simulink model "callGAMS"  (R2021b)
settings: Solver=ode1  StartTime=0.0  StopTime=20  FixedStep=1e-4  RelTol=1e-3
model workspace (MAT data in the model file):
  firstOrder = 60
  g2Max = 0
  runTime = 4
undefined symbols (not defined in the file or in its folder): c0, c1, D11, Delta, fg, G2gen, G3gen, G5gen, G6gen, G7gen, Iovc, l0, l1, Newton, r0, r1, Raphson, Rtpu, S1non, S2non, S3non, S5non, S6non, S7non, sigbuilder_block, tonvsc, Ts, Vhv, Vmv, w_pll, wc1, wdc1, wpq1, wsw1, Xtpu
libraries: simulink_extras x122, simulink x73, spsFirstOrderFilterLib x72, spsGroundLib x61, spsCurrentMeasurementLib x33, spsVoltageMeasurementLib x33, eeTransforms x24, spsabctoAlphaBetaZeroLib x12, spsControlledVoltageSourceLib x12, spsControlledCurrentSourceLib x12, spsPower3phPhasorLib x11, spsLoadFlowBusLib x9
(part 1 of 16)
Description:
  | Model of a simple control system for use iin training.
settings Model: SimulationMode=accelerator  PacingRate=0.100000  Creator=Paul Baracos  LastModifiedBy=oenoch
settings SolverCC: AlgebraicLoopSolver=TrustRegion
settings DataIOCC: LimitDataPoints=on  SaveOperatingPoint=on  SaveFormat=Array  SignalLoggingSaveFormat=ModelDataLogs  SaveOutput=off  SaveTime=off  ReturnWorkspaceOutputs=off  SignalLoggingName=sigsOut
settings OptimizationCC: BlockReduction=off  BooleanDataType=off  OptimizeBlockIOStorage=off  BufferReuse=off  GlobalBufferReuse=off  ExpressionFolding=off  LocalBlockOutputs=off  InitFltsAndDblsToZero=on  EfficientMapNaN2IntZero=off  LifeSpan=inf  OptimizeDataStoreBuffers=off  BusAssignmentInplaceUpdate=off
settings DebuggingCC: SaveWithParameterizedLinksMsg=none  UnderspecifiedInitializationDetection=Classic  MergeDetectMultiDrivingBlocksExec=none  SignalResolutionControl=TryResolveAllWithWarning  MultiTaskDSMMsg=warning  MultiTaskCondExecSysMsg=none  FcnCallInpInsideContextMsg=warning  UnconnectedInputMsg=none  UnconnectedOutputMsg=none  UnconnectedLineMsg=none  SFUnexpectedBacktrackingDiag=warning  SFNoUnconditionalDefaultTransitionDiag=warning  SFExecutionAtInitializationDiag=none  SFMachineParentedDataDiag=warning  ArithmeticOperatorsInVariantConditions=warning
settings HardwareCC: ProdBitPerPointer=32  ProdBitPerSizeT=32  ProdBitPerPtrDiffT=32  ProdLargestAtomicFloat=None  ProdIntDivRoundTo=Undefined  ProdEndianess=Unspecified  ProdWordSize=32  ProdHWDeviceType=32-bit Generic  TargetBitPerPointer=64  TargetBitPerSizeT=64  TargetBitPerPtrDiffT=64  TargetLongLongMode=on  TargetIntDivRoundTo=Zero  TargetEndianess=LittleEndian  TargetWordSize=64  TargetHWDeviceType=MATLAB Host  ProdEqTarget=off
settings ModelReferenceCC: PropagateSignalLabelsOutOfModel=off
settings SFSimCC: SimUseLocalCustomCode=off  CustomCodeUndefinedFunction=UseInterfaceOnly
settings CodeAppCC: MaxIdLength=128
settings GRTTargetCC: TargetLangStandard=C89/C90 (ANSI)  CombineOutputUpdateFcns=off  GRTInterface=on
settings ConfigComp: CovMetricSettings=dw  CovSaveCumulativeToWorkspaceVar=on  CovSaveSingleToWorkspaceVar=on  CovExternalEMLEnable=off

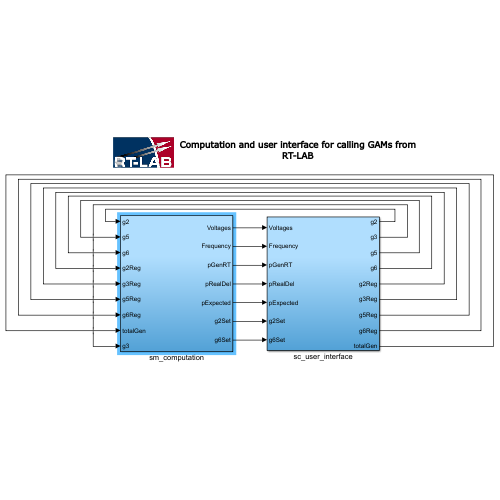
[thumbnail: Simulink's stored preview of the top-level diagram]
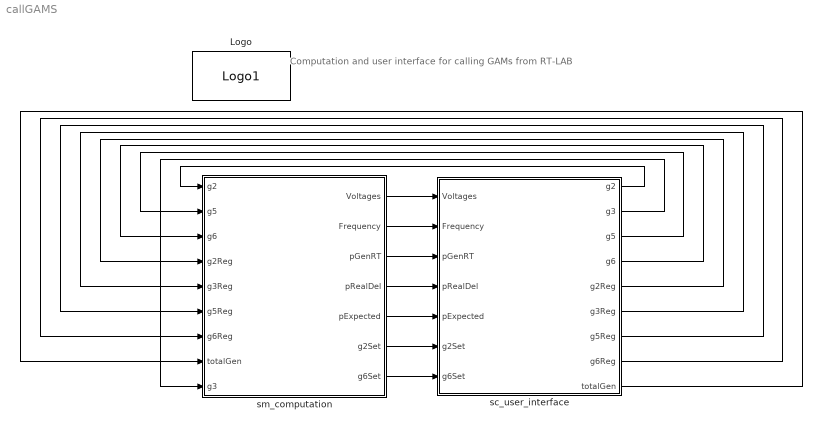
== system callGAMS ==
  note: Computation and user interface for calling GAMs from RT-LAB
  Logo : opal_lib/Logo1  vide=[]
  sc_user_interface : Subsystem
  sm_computation : Subsystem
  wires:
  sc_user_interface/1(g2) -> sm_computation/1(g2)
  sc_user_interface/2(g3) -> sm_computation/9(g3)
  sc_user_interface/3(g5) -> sm_computation/2(g5)
  sc_user_interface/4(g6) -> sm_computation/3(g6)
  sc_user_interface/5(g2Reg) -> sm_computation/4(g2Reg)
  sc_user_interface/6(g3Reg) -> sm_computation/5(g3Reg)
  sc_user_interface/7(g5Reg) -> sm_computation/6(g5Reg)
  sc_user_interface/8(g6Reg) -> sm_computation/7(g6Reg)
  sc_user_interface/9(totalGen) -> sm_computation/8(totalGen)
  sm_computation/1(Voltages) -> sc_user_interface/1(Voltages)
  sm_computation/2(Frequency) -> sc_user_interface/2(Frequency)
  sm_computation/3(pGenRT) -> sc_user_interface/3(pGenRT)
  sm_computation/4(pRealDel) -> sc_user_interface/4(pRealDel)
  sm_computation/5(pExpected) -> sc_user_interface/5(pExpected)
  sm_computation/6(g2Set) -> sc_user_interface/6(g2Set)
  sm_computation/7(g6Set) -> sc_user_interface/7(g6Set)

== system callGAMS/sc_user_interface ==
  note: Plots
  note: Input to the computation model
  note: Results from optimzation and dynamic model
  note: User interface: display acquisition signals and set control signals
  note: Real-time optimization
  Voltages : Inport
  Frequency : Inport  Port=2
  pGenRT : Inport  Port=3
  pRealDel : Inport  Port=4
  pExpected : Inport  Port=5
  g2Set : Inport  Port=6
  g6Set : Inport  Port=7
  Constant : Constant  OutMin=-10  OutMax=10
  Logo : opal_lib/Logo1  vide=[]
  OpComm : rtlab/OpComm  nbport=7  groupe_acq=1  subsys_rate=0  st=0  Synchronization=on  Interpolation=on  Threshold=1.0  Missed_Data=off  Sim_Time=off  Samples=off  dynSigOut=off  from_console=0  warning_done=off  writeOpCommFile=off  Offset=off
      settings: SourceProductName=RT-LAB
  Plots : Subsystem
  Pulse Generator : DiscretePulseGenerator  PulseType=Time based  Period=runTime  PulseWidth=5
  Pulse Generator1 : DiscretePulseGenerator  PulseType=Time based  Period=80  PulseWidth=5
  Real Time Redispatch Fn : Subsystem  TreatAsAtomicUnit=on
  Signal Builder : Subsystem  Tag=STV Subsys  Commented=on  LoadFcn=sigbuilder_block('load');  StartFcn=sigbuilder_block('start');  StopFcn=sigbuilder_block('stop');  ClipboardFcn=sigbuilder_block('clipboard');  mask(Sigbuilder block){tuvar=[0:10]}
      mask help: Simulink:masks:SigbuilderBlock_MD
      mask init:
      | if ~strcmp(get_param(bdroot(gcbh),'SimulationStatus'),'stopped') tuvar = sigbuilder_block('maskInit'); end
      settings: CopyFcn=sigbuilder_block('copy');  DeleteFcn=sigbuilder_block('delete');  ModelCloseFcn=sigbuilder_block('modelClose');  PreSaveFcn=sigbuilder_block('preSave');  PauseFcn=sigbuilder_block('pause');  ContinueFcn=sigbuilder_block('continue');  NameChangeFcn=sigbuilder_block('namechange');  OpenFcn=sigbuilder_block('open',[437.6 199.2 550.4 400 ]);  CloseFcn=sigbuilder_block('close');
      mask Display: plot(0, 0, 100, 100,[2, 2, 32, 32, 2], [68, 8, 8, 68, 68],[32, 2], [38, 38], [32, 19, 2],[53, 60, 44], [32, 17, 17, 2],[16, 16, 31, 31]);txt = getActiveGroup(gcbh);text(2, 100, txt,'verticalAlignment', 'top');
  TSO command : simulink/Math Operations/Slider Gain  gain=0  low=-50  high=50
  Triggered Subsystem : Subsystem  TreatAsAtomicUnit=on
  g2 : Outport
  g3 : Outport  Port=2
  g5 : Outport  Port=3
  g6 : Outport  Port=4
  g2Reg : Outport  Port=5
  g3Reg : Outport  Port=6
  g5Reg : Outport  Port=7
  g6Reg : Outport  Port=8
  totalGen : Outport  Port=9
  tag scope: freqs=global, g2Set=global, g6Set=global, voltages=global
  wires:
  TSO command/1 -> [tsoComm]
  Constant/1 -> TSO command/1
  [tsoComm] -> Real Time Redispatch Fn/1(tsoComm)
  Triggered Subsystem/1(Out1) -> Real Time Redispatch Fn/2(pGenRT)
  [pRealDel] -> Triggered Subsystem/2(In2)
  Triggered Subsystem/3(Output1) -> Real Time Redispatch Fn/4(gExpected)
  [pExpected] -> Triggered Subsystem/3(In3)
  Real Time Redispatch Fn/3(g5) -> g5/1, [g5]
  Triggered Subsystem/2(Output) -> Real Time Redispatch Fn/3(pPrev)
  Real Time Redispatch Fn/8(g6Reg) -> [g6Reg], g6Reg/1
  [pGenRT] -> Triggered Subsystem/1(In1)
  Real Time Redispatch Fn/2(g3) -> g3/1, [g3]
  Real Time Redispatch Fn/9(totalGen) -> [totalGen], totalGen/1
  Real Time Redispatch Fn/7(g5Reg) -> g5Reg/1
  Real Time Redispatch Fn/4(g6) -> g6/1, [g6]
  Real Time Redispatch Fn/6(g3Reg) -> g3Reg/1, [g3Reg]
  Pulse Generator/1 -> Real Time Redispatch Fn/Trigger
  Real Time Redispatch Fn/5(g2Reg) -> g2Reg/1, [g2Reg]
  Real Time Redispatch Fn/1(g2) -> g2/1, [g2]
  Pulse Generator1/1 -> Triggered Subsystem/Trigger
  Voltages/1 -> OpComm/1
  OpComm/1 -> [voltages]
  OpComm/2 -> [freqs]
  OpComm/3 -> [pGenRT]
  pGenRT/1 -> OpComm/3
  Frequency/1 -> OpComm/2
  pRealDel/1 -> OpComm/4
  pExpected/1 -> OpComm/5
  OpComm/4 -> [pRealDel]
  OpComm/5 -> [pExpected]
  g2Set/1 -> OpComm/6
  g6Set/1 -> OpComm/7
  OpComm/6 -> [g2Set]
  OpComm/7 -> [g6Set]

== system callGAMS/sm_computation ==
  note: Dynamic model
  note: Computation is done in this subsystem
  note: Results from optimzation and dynamic model
  g2 : Inport
  g5 : Inport  Port=2
  g6 : Inport  Port=3
  g2Reg : Inport  Port=4
  g3Reg : Inport  Port=5
  g5Reg : Inport  Port=6
  g6Reg : Inport  Port=7
  totalGen : Inport  Port=8
  g3 : Inport  Port=9
  B1 : Subsystem
  B2 : Subsystem
  B3 : Subsystem
  B4 : Subsystem
  B5 : Subsystem
  B6 : Subsystem
  B7 : Subsystem
  G1 : Subsystem
      mask Display:
      | disp('SG')
      | %x = [0:0.001:1];
      | %y = 0.2*sin(10*x) + 0.5;
      | %plot(x,y)
  G2 : Subsystem
  G2s : spsThreePhaseSourceLib/Three-Phase Source  Commented=on  InternalConnection=Yg  VoltagePhases=off  Voltage=(220000)*1.02346  PhaseAngle=-22.8275  Voltage_phases=[25e3 25e3 25e3]/sqrt(3)  PhaseAngles_phases=[0 -120 +120]  Frequency=fg  NonIdealSource=on  SpecifyImpedance=off  Resistance=Rtpu*(Vhv^2/S2non)  Inductance=Xtpu*(Vhv^2/S3non) * 1/(2*pi*fg)  ShortCircuitLevel=100e6  BaseVoltage=Vhv  XRratio=7  BusType=PQ  Pref=45000000  Qref=5000000  Prefabc=[10e3, 10e3, 10e3]  Qrefabc=[0, 0, 0]  Qmin=-inf  Qmax=inf
  G3 : Subsystem
  G3s : spsThreePhaseSourceLib/Three-Phase Source  Commented=on  InternalConnection=Yg  VoltagePhases=off  Voltage=(220000)*1.02196  PhaseAngle=-23.0407  Voltage_phases=[25e3 25e3 25e3]/sqrt(3)  PhaseAngles_phases=[0 -120 +120]  Frequency=fg  NonIdealSource=on  SpecifyImpedance=off  Resistance=Rtpu*(Vhv^2/S3non)  Inductance=Xtpu*(Vhv^2/S3non) * 1/(2*pi*fg)  ShortCircuitLevel=100e6  BaseVoltage=Vhv  XRratio=7  BusType=PQ  Pref=45000000  Qref=5000000  Prefabc=[10e3, 10e3, 10e3]  Qrefabc=[0, 0, 0]  Qmin=-inf  Qmax=inf
  G5 : Subsystem
  G5s : spsThreePhaseSourceLib/Three-Phase Source  Commented=on  InternalConnection=Yg  VoltagePhases=off  Voltage=(220000)*1.02214  PhaseAngle=-22.9944  Voltage_phases=[25e3 25e3 25e3]/sqrt(3)  PhaseAngles_phases=[0 -120 +120]  Frequency=fg  NonIdealSource=on  SpecifyImpedance=off  Resistance=Rtpu*(Vhv^2/S5non)  Inductance=Xtpu*(Vhv^2/S5non) * 1/(2*pi*fg)  ShortCircuitLevel=100e6  BaseVoltage=Vhv  XRratio=7  BusType=PQ  Pref=45000000  Qref=5000000  Prefabc=[10e3, 10e3, 10e3]  Qrefabc=[0, 0, 0]  Qmin=-inf  Qmax=inf
  G6 : Subsystem
  G6s : spsThreePhaseSourceLib/Three-Phase Source  Commented=on  InternalConnection=Yg  VoltagePhases=off  Voltage=(220000)*1.02275  PhaseAngle=-22.9111  Voltage_phases=[25e3 25e3 25e3]/sqrt(3)  PhaseAngles_phases=[0 -120 +120]  Frequency=fg  NonIdealSource=on  SpecifyImpedance=off  Resistance=Rtpu*(Vhv^2/S6non)  Inductance=Xtpu*(Vhv^2/S6non) * 1/(2*pi*fg)  ShortCircuitLevel=100e6  BaseVoltage=Vhv  XRratio=7  BusType=PQ  Pref=45000000  Qref=5000000  Prefabc=[10e3, 10e3, 10e3]  Qrefabc=[0, 0, 0]  Qmin=-inf  Qmax=inf
  G7 : Subsystem
      mask Display:
      | disp('SG')
      | %x = [0:0.001:1];
      | %y = 0.2*sin(10*x) + 0.5;
      | %plot(x,y)
  Logo : opal_lib/Logo1  vide=[]
  Measurements EMT : Subsystem  Commented=on
  Measurements Phasor : Subsystem
  OpComm : rtlab/OpComm  nbport=9  groupe_acq=1  subsys_rate=0  st=0  Synchronization=on  Interpolation=on  Threshold=1.0  Missed_Data=off  Sim_Time=off  Samples=off  dynSigOut=off  from_console=1  warning_done=off  writeOpCommFile=off  Offset=off
      settings: SourceProductName=RT-LAB
  Three-Phase PI Section Line{1,3,7,10} (4 alike) : spsThreePhasePISectionLineLib/Three-Phase PI Section Line  LConnTagsString=a|b|c  RConnTagsString=A|B|C  Length=20  Frequency=fg  Resistances=[r1 r0]  Inductances="[l1  l0]"  Capacitances=[c1 c0]
  Three-Phase PI Section Line2 : spsThreePhasePISectionLineLib/Three-Phase PI Section Line  LConnTagsString=a|b|c  RConnTagsString=A|B|C  Length=40  Frequency=fg  Resistances=[r1 r0]  Inductances="[l1  l0]"  Capacitances=[c1 c0]
  Three-Phase PI Section Line4 : spsThreePhasePISectionLineLib/Three-Phase PI Section Line  LConnTagsString=a|b|c  RConnTagsString=A|B|C  Length=10  Frequency=fg  Resistances=[r1 r0]  Inductances="[l1  l0]"  Capacitances=[c1 c0]
  Three-Phase PI Section Line5 : spsThreePhasePISectionLineLib/Three-Phase PI Section Line  LConnTagsString=a|b|c  RConnTagsString=A|B|C  Length=30  Frequency=fg  Resistances=[r1 r0]  Inductances="[l1  l0]"  Capacitances=[c1 c0]
  Three-Phase PI Section Line9 : spsThreePhasePISectionLineLib/Three-Phase PI Section Line  LConnTagsString=a|b|c  RConnTagsString=A|B|C  Length=10  Frequency=fg  Resistances=[r1 r0]  Inductances="[l1  l0]"  Capacitances=[c1 c0]
  Three-Phase Parallel RLC Load1 : spsThreePhaseParallelRLCLoadLib/Three-Phase Parallel RLC Load  LConnTagsString=A|B|C  Configuration=Y (grounded)  NominalVoltage=Vhv  Vabc=[1e3 1e3 1e3]  Vabcp=[1e3 1e3 1e3]  NominalFrequency=fg  UnbalancedPower=off  ActivePower=81750000  InductivePower=10196203.4628  CapacitivePower=0  Pabc=[10e3 9e3 11e3]  QLabc=[100 90 110]  QCabc=[100 90 110]  Pabcp=[10e3 9e3 11e3]  QLabcp=[100 90 110]  QCabcp=[100 90 110]  Measurements=None  LoadType=constant Z
  Three-Phase Parallel RLC Load2 : spsThreePhaseParallelRLCLoadLib/Three-Phase Parallel RLC Load  LConnTagsString=A|B|C  Configuration=Y (grounded)  NominalVoltage=Vhv  Vabc=[1e3 1e3 1e3]  Vabcp=[1e3 1e3 1e3]  NominalFrequency=fg  UnbalancedPower=off  ActivePower=115375000  InductivePower=20395570.7066  CapacitivePower=0  Pabc=[10e3 9e3 11e3]  QLabc=[100 90 110]  QCabc=[100 90 110]  Pabcp=[10e3 9e3 11e3]  QLabcp=[100 90 110]  QCabcp=[100 90 110]  Measurements=None  LoadType=constant Z
  Three-Phase Parallel RLC Load3 : spsThreePhaseParallelRLCLoadLib/Three-Phase Parallel RLC Load  LConnTagsString=A|B|C  Configuration=Y (grounded)  NominalVoltage=Vhv  Vabc=[1e3 1e3 1e3]  Vabcp=[1e3 1e3 1e3]  NominalFrequency=fg  UnbalancedPower=off  ActivePower=47250000  InductivePower=5398734.4876  CapacitivePower=0  Pabc=[10e3 9e3 11e3]  QLabc=[100 90 110]  QCabc=[100 90 110]  Pabcp=[10e3 9e3 11e3]  QLabcp=[100 90 110]  QCabcp=[100 90 110]  Measurements=None  LoadType=constant Z
  Three-Phase Parallel RLC Load6 : spsThreePhaseParallelRLCLoadLib/Three-Phase Parallel RLC Load  LConnTagsString=A|B|C  Configuration=Y (grounded)  NominalVoltage=Vhv  Vabc=[1e3 1e3 1e3]  Vabcp=[1e3 1e3 1e3]  NominalFrequency=fg  UnbalancedPower=off  ActivePower=47250000  InductivePower=10398734.4876  CapacitivePower=0  Pabc=[10e3 9e3 11e3]  QLabc=[100 90 110]  QCabc=[100 90 110]  Pabcp=[10e3 9e3 11e3]  QLabcp=[100 90 110]  QCabcp=[100 90 110]  Measurements=None  LoadType=constant Z
  Three-Phase Parallel RLC Load7 : spsThreePhaseParallelRLCLoadLib/Three-Phase Parallel RLC Load  LConnTagsString=A|B|C  Configuration=Y (grounded)  NominalVoltage=Vhv  Vabc=[1e3 1e3 1e3]  Vabcp=[1e3 1e3 1e3]  NominalFrequency=fg  UnbalancedPower=off  ActivePower=20875000  InductivePower=5598101.7314  CapacitivePower=0  Pabc=[10e3 9e3 11e3]  QLabc=[100 90 110]  QCabc=[100 90 110]  Pabcp=[10e3 9e3 11e3]  QLabcp=[100 90 110]  QCabcp=[100 90 110]  Measurements=None  LoadType=constant Z
  powergui : spspowerguiLib/powergui  Priority=1  SimulationMode=Phasor  SampleTime=50e-6  frequency=fg  Iterations=50  frequencyindice=50  Pbase=100e6  ErrMax=0.0001  UnitsV=kV  UnitsW=MW  buscounter=0  FunctionMessages=off  echomessages=off  EnableUseOfTLC=off  CurrentSourceSwitches=off  DisableSnubberDevices=off  DisableRonSwitches=off  DisableVfSwitches=off  DisplayEquations=off  AutomaticDiscreteSolvers=off  SolverType=Tustin/Backward Euler (TBE)  Interpol=off  ExternalGateDelay=off  methode=off  Ts=100  x0status=blocks  SPID=on  SwTol=0  HookPort=off  NonlinearTolerance=1e-4  nMaxIteration=100  ContinueOnMaxIteration=off  RestoreLinks=warning  ResistiveCurrentMeasurement=off  Frange=[0:2:500]  Ylog=off  Xlog=on  ShowGrid=off  save=off  variable=ZData  structure=0  ZoomFFT=off  StartTime=0.0  cycles=1  DisplayStyle=1  fundamental=60  FreqAxis=off  MaxFrequency=1000  frequencyindicesteady=1  RmsSteady=1  display=off
  Voltages : Outport
  Frequency : Outport  Port=2
  pGenRT : Outport  Port=3
  pRealDel : Outport  Port=4  VectorParamsAs1DForOutWhenUnconnected=off
  pExpected : Outport  Port=5  VectorParamsAs1DForOutWhenUnconnected=off
  g2Set : Outport  Port=6  VectorParamsAs1DForOutWhenUnconnected=off
  g6Set : Outport  Port=7  VectorParamsAs1DForOutWhenUnconnected=off
  tag scope: g2=global, g2Reg=global, g3=global, g3Reg=global, g5=global, g5Reg=global, g6=global, g6Reg=global, totalGen=global
  wires:
  Measurements Phasor/1(Voltages) -> Voltages/1
  Measurements Phasor/2(Frequency) -> Frequency/1
  totalGen/1 -> OpComm/9
  g6Reg/1 -> OpComm/8
  g5Reg/1 -> OpComm/7
  g3Reg/1 -> OpComm/6
  g2Reg/1 -> OpComm/5
  g6/1 -> OpComm/4
  g5/1 -> OpComm/3
  g2/1 -> OpComm/1
  g3/1 -> OpComm/2
  OpComm/1 -> [g2]
  OpComm/5 -> [g2Reg]
  OpComm/2 -> [g3]
  OpComm/3 -> [g5]
  OpComm/4 -> [g6]
  OpComm/6 -> [g3Reg]
  OpComm/7 -> [g5Reg]
  OpComm/8 -> [g6Reg]
  OpComm/9 -> [totalGen]
  Measurements Phasor/3(pGenRT) -> pGenRT/1
  Measurements Phasor/4(pRealDel) -> pRealDel/1
  Measurements Phasor/5(pExpected) -> pExpected/1
  G2/1(Output) -> g2Set/1
  G6/1(Output) -> g6Set/1
  connections:
  Three-Phase PI Section Line1/LConn1 -- B2/RConn1 -- Three-Phase PI Section Line7/LConn1
  B5/RConn3 -- Three-Phase PI Section Line5/LConn3 -- Three-Phase PI Section Line7/RConn3 -- Three-Phase PI Section Line3/LConn3 -- Three-Phase PI Section Line4/LConn3 -- Three-Phase Parallel RLC Load2/LConn3
  Three-Phase Parallel RLC Load7/LConn1 -- Three-Phase PI Section Line10/RConn1 -- Three-Phase PI Section Line3/RConn1 -- B6/LConn1
  Three-Phase Parallel RLC Load3/LConn1 -- B7/LConn1 -- Three-Phase PI Section Line5/RConn1
  B4/RConn1 -- Three-Phase PI Section Line9/LConn1 -- Three-Phase PI Section Line10/LConn1 -- Three-Phase PI Section Line2/RConn1
  Three-Phase PI Section Line9/RConn2 -- B3/LConn2 -- Three-Phase Parallel RLC Load6/LConn2
  Three-Phase Parallel RLC Load7/LConn2 -- Three-Phase PI Section Line10/RConn2 -- Three-Phase PI Section Line3/RConn2 -- B6/LConn2
  Three-Phase PI Section Line9/RConn1 -- B3/LConn1 -- Three-Phase Parallel RLC Load6/LConn1
  Three-Phase Parallel RLC Load3/LConn3 -- B7/LConn3 -- Three-Phase PI Section Line5/RConn3
  B6/RConn2 -- G6s/RConn2 -- G6/RConn2
  B5/RConn1 -- Three-Phase PI Section Line5/LConn1 -- Three-Phase PI Section Line7/RConn1 -- Three-Phase PI Section Line3/LConn1 -- Three-Phase PI Section Line4/LConn1 -- Three-Phase Parallel RLC Load2/LConn1
  Three-Phase PI Section Line1/LConn3 -- B2/RConn3 -- Three-Phase PI Section Line7/LConn3
  B3/RConn2 -- G3s/RConn2 -- G3/RConn2
  B5/RConn2 -- Three-Phase PI Section Line5/LConn2 -- Three-Phase PI Section Line7/RConn2 -- Three-Phase PI Section Line3/LConn2 -- Three-Phase PI Section Line4/LConn2 -- Three-Phase Parallel RLC Load2/LConn2
  B6/RConn3 -- G6s/RConn3 -- G6/RConn3
  Three-Phase Parallel RLC Load1/LConn2 -- B4/LConn2 -- Three-Phase PI Section Line4/RConn2 -- Three-Phase PI Section Line1/RConn2
  B3/RConn1 -- G3s/RConn1 -- G3/RConn1
  B3/RConn3 -- G3s/RConn3 -- G3/RConn3
  Three-Phase Parallel RLC Load1/LConn1 -- B4/LConn1 -- Three-Phase PI Section Line4/RConn1 -- Three-Phase PI Section Line1/RConn1
  Three-Phase Parallel RLC Load3/LConn2 -- B7/LConn2 -- Three-Phase PI Section Line5/RConn2
  Three-Phase PI Section Line9/RConn3 -- B3/LConn3 -- Three-Phase Parallel RLC Load6/LConn3
  B6/RConn1 -- G6s/RConn1 -- G6/RConn1
  Three-Phase PI Section Line1/LConn2 -- B2/RConn2 -- Three-Phase PI Section Line7/LConn2
  B2/LConn3 -- G2s/RConn3 -- G2/RConn3
  B2/LConn1 -- G2s/RConn1 -- G2/RConn1
  Three-Phase Parallel RLC Load7/LConn3 -- Three-Phase PI Section Line10/RConn3 -- Three-Phase PI Section Line3/RConn3 -- B6/LConn3
  Three-Phase Parallel RLC Load1/LConn3 -- B4/LConn3 -- Three-Phase PI Section Line4/RConn3 -- Three-Phase PI Section Line1/RConn3
  Three-Phase PI Section Line2/LConn3 -- B1/RConn3
  Three-Phase PI Section Line2/LConn1 -- B1/RConn1
  G1/RConn1 -- B1/LConn1
  G1/RConn2 -- B1/LConn2
  Three-Phase PI Section Line2/LConn2 -- B1/RConn2
  G1/RConn3 -- B1/LConn3
  G7/RConn1 -- B7/RConn1
  G7/RConn2 -- B7/RConn2
  G7/RConn3 -- B7/RConn3
  B4/RConn3 -- Three-Phase PI Section Line10/LConn3 -- Three-Phase PI Section Line9/LConn3 -- Three-Phase PI Section Line2/RConn3
  B4/RConn2 -- Three-Phase PI Section Line2/RConn2 -- Three-Phase PI Section Line9/LConn2 -- Three-Phase PI Section Line10/LConn2
  G5s/RConn3 -- G5/RConn3 -- B5/LConn3
  G5/RConn1 -- G5s/RConn1 -- B5/LConn1
  G2s/RConn2 -- B2/LConn2 -- G2/RConn2
  G5/RConn2 -- B5/LConn2 -- G5s/RConn2

== system callGAMS/sc_user_interface/Plots ==
  note: Multiple commands
  note: System parameters
  note: Individual active power generation and regulation of VPP units
  note: Total active power generation from Pset,
      | units and dynamic model
  All o/p scope : Scope
  Frequency scope : Scope
  From10 : From  Commented=on  GotoTag=g2Set
  From12 : From  Commented=on  GotoTag=g3Set
  From13 : From  Commented=on  GotoTag=g5Set
  From29 : From  Commented=on  GotoTag=g6Set
  Gain : Gain  Gain=1/100
  Gain1 : Gain  Gain=1/100
  Gain2 : Gain  Gain=1e6
  Generation and Regulation scope : Scope
  Goto3 : Goto  Commented=on  GotoTag=pSet  TagVisibility=global
  Integrator : Integrator  InitialCondition=S2non*G2gen
  Integrator1 : Integrator  InitialCondition=S6non*G6gen
  Mux : Mux  Inputs=2
  Mux1 : Mux  Inputs=8
  Mux10 : Mux  Inputs=2
  Mux6 : Mux  Commented=on
  Mux8 : Mux
  Mux9 : Mux
  Power scope : Scope
  Sum : Sum  Inputs=|+-
  Sum of Elements : Sum  Commented=on  Inputs=+
  Sum1 : Sum  Inputs=|+-
  Sum2 : Sum  Inputs=+-+-
  To Workspace : ToWorkspace  VariableName=pGoutWpp  SaveFormat=Structure With Time  SampleTime=-1
  To Workspace1 : ToWorkspace  VariableName=pGoutPv  SaveFormat=Structure With Time  SampleTime=-1
  To Workspace2 : ToWorkspace  VariableName=pMultiple  SaveFormat=Structure With Time  SampleTime=-1
  Voltage scope : Scope
  g2 scope1 : Scope  NumInputPorts=2
  g2 scope2 : Scope
  wires:
  [g2] -> Mux1/1
  [g5P] -> Mux1/3
  [g6P] -> Mux1/4
  [g2RegP] -> Mux1/5
  [pGenRT] -> Power scope/1
  [voltages] -> Voltage scope/1
  [freqs] -> Frequency scope/1
  From10/1 -> Mux6/3
  From12/1 -> Mux6/2
  [pSet] -> Mux/1  "pSet"
  From13/1 -> Mux6/1
  Mux/1 -> All o/p scope/1
  Mux1/1 -> Generation and Regulation scope/1
  [activePowerSum] -> Mux/2  "dynamic"
  [g5RegP] -> Mux1/7
  [g6RegP] -> Mux1/8
  From29/1 -> Mux6/4
  Mux6/1 -> Goto3/1, Sum of Elements/1
  Mux8/1 -> g2 scope1/1, To Workspace/1
  [g2Actual] -> Mux8/1  "Normal offer"
  [g2Set] -> Mux8/3  "gSet"
  Gain/1 -> Integrator/1
  Sum/1 -> Gain/1
  Integrator/1 -> Sum/2, Mux8/4  "First order 100secs"
  [g2Expected] -> Mux8/2, Sum/1  "Ex s"
  [g6Expected] -> Mux9/2, Sum1/1
  Sum1/1 -> Gain1/1
  Gain1/1 -> Integrator1/1
  [g6Actual] -> Mux9/1
  Integrator1/1 -> Mux9/4, Sum1/2  "First order 100secs"
  [g6Set] -> Mux9/3
  Mux9/1 -> g2 scope1/2, To Workspace1/1
  [tsoComm] -> Gain2/1
  Mux10/1 -> g2 scope2/1, To Workspace2/1
  [g2Set] -> Sum2/1  "gSet"
  [g6Set] -> Sum2/3  "gSet"
  [g2Actual] -> Sum2/2
  [g6Actual] -> Sum2/4
  Sum2/1 -> [rEff]
  [rEff] -> Mux10/2
  Gain2/1 -> Mux10/1

== system callGAMS/sc_user_interface/Real Time Redispatch Fn ==
  tsoComm : Inport
  pGenRT : Inport  Port=2
  pPrev : Inport  Port=3
  gExpected : Inport  Port=4
  Trigger : TriggerPort  VariantControl=(inherit)
  MATLAB Function : MATLAB Function  TreatAsAtomicUnit=on
  g2 : Outport
  g3 : Outport  Port=2
  g5 : Outport  Port=3
  g6 : Outport  Port=4
  g2Reg : Outport  Port=5
  g3Reg : Outport  Port=6
  g5Reg : Outport  Port=7
  g6Reg : Outport  Port=8
  totalGen : Outport  Port=9
  wires:
  MATLAB Function/7(g5Reg) -> g5Reg/1
  MATLAB Function/6(g3Reg) -> g3Reg/1
  MATLAB Function/1(g2) -> g2/1
  MATLAB Function/4(g6) -> g6/1
  MATLAB Function/5(g2Reg) -> g2Reg/1
  MATLAB Function/3(g5) -> g5/1
  MATLAB Function/2(g3) -> g3/1
  tsoComm/1 -> MATLAB Function/1(tsoComm)
  pGenRT/1 -> MATLAB Function/2(pGenRT)
  pPrev/1 -> MATLAB Function/3(pPrev)
  gExpected/1 -> MATLAB Function/4(pExpected)
  MATLAB Function/8(g6Reg) -> g6Reg/1
  MATLAB Function/9(totalGen) -> totalGen/1

== system callGAMS/sc_user_interface/Signal Builder ==
  Demux : Demux  Tag=STV Demux  Outputs=1
      settings: DisplayOption=none
  FromWs : FromWorkspace  Tag=STV FromWs  VariableName=tuvar
      SigBuilderData=|
      | common.afterFinalStr = 'Extrapolate'
      | common.sampleTime = 0
      | dataSet.timeRange = [0 10]
      | dataSet.name = 'Group 1'
      | sbobj.Groups.Name = 'Group 1'
      | sbobj.Groups.Signals.Name = 'Signal 1'
      | sbobj.Groups.Signals.XData = [0 4 4 6 6 10]
      | sbobj.Groups.Signals.YData = [0 0 1 1 0 0]
  Signal 1 : Outport  Tag=STV Outport
  wires:
  Demux/1 -> Signal 1/1
  FromWs/1 -> Demux/1

== system callGAMS/sc_user_interface/Triggered Subsystem ==
  In1 : Inport  LatchByDelayingOutsideSignal=on
  In2 : Inport  Port=2  LatchByDelayingOutsideSignal=on
  In3 : Inport  Port=3  LatchByDelayingOutsideSignal=on
  Trigger : TriggerPort  VariantControl=(inherit)
  Out1 : Outport
  Output : Outport  Port=2
  Output1 : Outport  Port=3
  wires:
  In1/1 -> Out1/1
  In2/1 -> Output/1
  In3/1 -> Output1/1

== system callGAMS/sm_computation/B1 ==
  Current Measurement1 : spsCurrentMeasurementLib/Current Measurement  PhasorSimulation=on  OutputType=Complex  PSBequivalent=0
  Current Measurement2 : spsCurrentMeasurementLib/Current Measurement  PhasorSimulation=on  OutputType=Complex  PSBequivalent=0
  Current Measurement3 : spsCurrentMeasurementLib/Current Measurement  PhasorSimulation=on  OutputType=Complex  PSBequivalent=0
  Gain : Gain
  Gain1 : Gain
  Ground1 : spsGroundLib/Ground  LConnTagsString=a
  Ground2 : spsGroundLib/Ground  LConnTagsString=a
  Ground3 : spsGroundLib/Ground  LConnTagsString=a
  Load Flow Bus1 : spsLoadFlowBusLib/Load Flow Bus  LConnTagsString=a  Phases=single  Connectors=on one side  ID=B1  Vbase=Vhv  Vref=1  Vangle=0  VLF=1  VLFb=1  VLFc=1  angleLF=-30.01  angleLFb=0  angleLFc=0
      settings: SourceProductBaseCode=PS
  Mux : Mux  Inputs=3
  Mux1 : Mux  Inputs=3
  Voltage Measurement1 : spsVoltageMeasurementLib/Voltage Measurement  PhasorSimulation=on  OutputType=Complex  PSBequivalent=0
  Voltage Measurement2 : spsVoltageMeasurementLib/Voltage Measurement  PhasorSimulation=on  OutputType=Complex  PSBequivalent=0
  Voltage Measurement3 : spsVoltageMeasurementLib/Voltage Measurement  PhasorSimulation=on  OutputType=Complex  PSBequivalent=0
  A : PMIOPort  Side=Left
  B : PMIOPort  Port=2  Side=Left
  C : PMIOPort  Port=3  Side=Left
  a : PMIOPort  Port=4  Side=Right
  b : PMIOPort  Port=5  Side=Right
  c : PMIOPort  Port=6  Side=Right
  tag scope: Ig1=global, Vg1=global
  wires:
  Voltage Measurement2/1 -> Mux/3
  Voltage Measurement1/1 -> Mux/2
  Voltage Measurement3/1 -> Mux/1
  Current Measurement3/1 -> Mux1/1
  Current Measurement1/1 -> Mux1/2
  Current Measurement2/1 -> Mux1/3
  Mux/1 -> Gain/1
  Gain/1 -> [Vg1]
  Mux1/1 -> Gain1/1
  Gain1/1 -> [Ig1]
  connections:
  Current Measurement3/RConn1 -- a/RConn1
  B/RConn1 -- Current Measurement1/LConn1 -- Voltage Measurement1/LConn1
  C/RConn1 -- Current Measurement2/LConn1 -- Voltage Measurement2/LConn1
  Current Measurement3/LConn1 -- Voltage Measurement3/LConn1 -- Load Flow Bus1/LConn1 -- A/RConn1
  Current Measurement1/RConn1 -- b/RConn1
  Current Measurement2/RConn1 -- c/RConn1
  Ground3/LConn1 -- Voltage Measurement3/LConn2
  Ground1/LConn1 -- Voltage Measurement1/LConn2
  Ground2/LConn1 -- Voltage Measurement2/LConn2

== system callGAMS/sm_computation/B2 ==
  Current Measurement1 : spsCurrentMeasurementLib/Current Measurement  PhasorSimulation=on  OutputType=Complex  PSBequivalent=0
  Current Measurement2 : spsCurrentMeasurementLib/Current Measurement  PhasorSimulation=on  OutputType=Complex  PSBequivalent=0
  Current Measurement3 : spsCurrentMeasurementLib/Current Measurement  PhasorSimulation=on  OutputType=Complex  PSBequivalent=0
  Gain : Gain
  Gain1 : Gain
  Ground1 : spsGroundLib/Ground  LConnTagsString=a
  Ground2 : spsGroundLib/Ground  LConnTagsString=a
  Ground3 : spsGroundLib/Ground  LConnTagsString=a
  Load Flow Bus1 : spsLoadFlowBusLib/Load Flow Bus  LConnTagsString=a  Phases=single  Connectors=on one side  ID=B2  Vbase=Vhv  Vref=1  Vangle=0  VLF=0.9961  VLFb=1  VLFc=1  angleLF=-30.42  angleLFb=0  angleLFc=0
      settings: SourceProductBaseCode=PS
  Mux : Mux  Inputs=3
  Mux1 : Mux  Inputs=3
  Voltage Measurement1 : spsVoltageMeasurementLib/Voltage Measurement  PhasorSimulation=on  OutputType=Complex  PSBequivalent=0
  Voltage Measurement2 : spsVoltageMeasurementLib/Voltage Measurement  PhasorSimulation=on  OutputType=Complex  PSBequivalent=0
  Voltage Measurement3 : spsVoltageMeasurementLib/Voltage Measurement  PhasorSimulation=on  OutputType=Complex  PSBequivalent=0
  A : PMIOPort  Side=Left
  B : PMIOPort  Port=2  Side=Left
  C : PMIOPort  Port=3  Side=Left
  a : PMIOPort  Port=4  Side=Right
  b : PMIOPort  Port=5  Side=Right
  c : PMIOPort  Port=6  Side=Right
  tag scope: Ig2=global, Vg2=global
  wires:
  Voltage Measurement2/1 -> Mux/3
  Voltage Measurement1/1 -> Mux/2
  Voltage Measurement3/1 -> Mux/1
  Current Measurement3/1 -> Mux1/1
  Current Measurement1/1 -> Mux1/2
  Current Measurement2/1 -> Mux1/3
  Mux/1 -> Gain/1
  Gain/1 -> [Vg2]
  Mux1/1 -> Gain1/1
  Gain1/1 -> [Ig2]
  connections:
  Current Measurement3/RConn1 -- a/RConn1
  Voltage Measurement1/LConn1 -- B/RConn1 -- Current Measurement1/LConn1
  Voltage Measurement2/LConn1 -- C/RConn1 -- Current Measurement2/LConn1
  Voltage Measurement3/LConn1 -- Load Flow Bus1/LConn1 -- A/RConn1 -- Current Measurement3/LConn1
  Current Measurement1/RConn1 -- b/RConn1
  Current Measurement2/RConn1 -- c/RConn1
  Ground3/LConn1 -- Voltage Measurement3/LConn2
  Ground1/LConn1 -- Voltage Measurement1/LConn2
  Ground2/LConn1 -- Voltage Measurement2/LConn2

== system callGAMS/sm_computation/B3 ==
  Current Measurement1 : spsCurrentMeasurementLib/Current Measurement  PhasorSimulation=on  OutputType=Complex  PSBequivalent=0
  Current Measurement2 : spsCurrentMeasurementLib/Current Measurement  PhasorSimulation=on  OutputType=Complex  PSBequivalent=0
  Current Measurement3 : spsCurrentMeasurementLib/Current Measurement  PhasorSimulation=on  OutputType=Complex  PSBequivalent=0
  Gain : Gain
  Gain1 : Gain
  Ground1 : spsGroundLib/Ground  LConnTagsString=a
  Ground2 : spsGroundLib/Ground  LConnTagsString=a
  Ground3 : spsGroundLib/Ground  LConnTagsString=a
  Load Flow Bus1 : spsLoadFlowBusLib/Load Flow Bus  LConnTagsString=a  Phases=single  Connectors=on one side  ID=B3  Vbase=Vhv  Vref=1  Vangle=0  VLF=0.9945  VLFb=1  VLFc=1  angleLF=-30.65  angleLFb=0  angleLFc=0
      settings: SourceProductBaseCode=PS
  Mux : Mux  Inputs=3
  Mux1 : Mux  Inputs=3
  Voltage Measurement1 : spsVoltageMeasurementLib/Voltage Measurement  PhasorSimulation=on  OutputType=Complex  PSBequivalent=0
  Voltage Measurement2 : spsVoltageMeasurementLib/Voltage Measurement  PhasorSimulation=on  OutputType=Complex  PSBequivalent=0
  Voltage Measurement3 : spsVoltageMeasurementLib/Voltage Measurement  PhasorSimulation=on  OutputType=Complex  PSBequivalent=0
  A : PMIOPort  Side=Left
  B : PMIOPort  Port=2  Side=Left
  C : PMIOPort  Port=3  Side=Left
  a : PMIOPort  Port=4  Side=Right
  b : PMIOPort  Port=5  Side=Right
  c : PMIOPort  Port=6  Side=Right
  tag scope: Ig3=global, Vg3=global
  wires:
  Voltage Measurement2/1 -> Mux/3
  Voltage Measurement1/1 -> Mux/2
  Voltage Measurement3/1 -> Mux/1
  Current Measurement3/1 -> Mux1/1
  Current Measurement1/1 -> Mux1/2
  Current Measurement2/1 -> Mux1/3
  Mux/1 -> Gain/1
  Gain/1 -> [Vg3]
  Mux1/1 -> Gain1/1
  Gain1/1 -> [Ig3]
  connections:
  Current Measurement3/RConn1 -- a/RConn1
  Voltage Measurement1/LConn1 -- B/RConn1 -- Current Measurement1/LConn1
  Voltage Measurement2/LConn1 -- C/RConn1 -- Current Measurement2/LConn1
  Voltage Measurement3/LConn1 -- Load Flow Bus1/LConn1 -- A/RConn1 -- Current Measurement3/LConn1
  Current Measurement1/RConn1 -- b/RConn1
  Current Measurement2/RConn1 -- c/RConn1
  Ground3/LConn1 -- Voltage Measurement3/LConn2
  Ground1/LConn1 -- Voltage Measurement1/LConn2
  Ground2/LConn1 -- Voltage Measurement2/LConn2

== system callGAMS/sm_computation/B4 ==
  Current Measurement1 : spsCurrentMeasurementLib/Current Measurement  PhasorSimulation=on  OutputType=Complex  PSBequivalent=0
  Current Measurement2 : spsCurrentMeasurementLib/Current Measurement  PhasorSimulation=on  OutputType=Complex  PSBequivalent=0
  Current Measurement3 : spsCurrentMeasurementLib/Current Measurement  PhasorSimulation=on  OutputType=Complex  PSBequivalent=0
  Gain : Gain
  Gain1 : Gain
  Ground1 : spsGroundLib/Ground  LConnTagsString=a
  Ground2 : spsGroundLib/Ground  LConnTagsString=a
  Ground3 : spsGroundLib/Ground  LConnTagsString=a
  Load Flow Bus1 : spsLoadFlowBusLib/Load Flow Bus  LConnTagsString=a  Phases=single  Connectors=on one side  ID=B4  Vbase=Vhv  Vref=1  Vangle=0  VLF=0.9949  VLFb=1  VLFc=1  angleLF=-30.65  angleLFb=0  angleLFc=0
      settings: SourceProductBaseCode=PS
  Mux : Mux  Inputs=3
  Mux1 : Mux  Inputs=3
  Voltage Measurement1 : spsVoltageMeasurementLib/Voltage Measurement  PhasorSimulation=on  OutputType=Complex  PSBequivalent=0
  Voltage Measurement2 : spsVoltageMeasurementLib/Voltage Measurement  PhasorSimulation=on  OutputType=Complex  PSBequivalent=0
  Voltage Measurement3 : spsVoltageMeasurementLib/Voltage Measurement  PhasorSimulation=on  OutputType=Complex  PSBequivalent=0
  A : PMIOPort  Side=Left
  B : PMIOPort  Port=2  Side=Left
  C : PMIOPort  Port=3  Side=Left
  a : PMIOPort  Port=4  Side=Right
  b : PMIOPort  Port=5  Side=Right
  c : PMIOPort  Port=6  Side=Right
  tag scope: Ig4=global, Vg4=global
  wires:
  Voltage Measurement2/1 -> Mux/3
  Voltage Measurement1/1 -> Mux/2
  Voltage Measurement3/1 -> Mux/1
  Current Measurement3/1 -> Mux1/1
  Current Measurement1/1 -> Mux1/2
  Current Measurement2/1 -> Mux1/3
  Mux/1 -> Gain/1
  Gain/1 -> [Vg4]
  Mux1/1 -> Gain1/1
  Gain1/1 -> [Ig4]
  connections:
  Current Measurement3/RConn1 -- a/RConn1
  Voltage Measurement1/LConn1 -- B/RConn1 -- Current Measurement1/LConn1
  Voltage Measurement2/LConn1 -- C/RConn1 -- Current Measurement2/LConn1
  Voltage Measurement3/LConn1 -- Load Flow Bus1/LConn1 -- A/RConn1 -- Current Measurement3/LConn1
  Current Measurement1/RConn1 -- b/RConn1
  Current Measurement2/RConn1 -- c/RConn1
  Ground3/LConn1 -- Voltage Measurement3/LConn2
  Ground1/LConn1 -- Voltage Measurement1/LConn2
  Ground2/LConn1 -- Voltage Measurement2/LConn2

== system callGAMS/sm_computation/B5 ==
  Current Measurement1 : spsCurrentMeasurementLib/Current Measurement  PhasorSimulation=on  OutputType=Complex  PSBequivalent=0
  Current Measurement2 : spsCurrentMeasurementLib/Current Measurement  PhasorSimulation=on  OutputType=Complex  PSBequivalent=0
  Current Measurement3 : spsCurrentMeasurementLib/Current Measurement  PhasorSimulation=on  OutputType=Complex  PSBequivalent=0
  Gain : Gain
  Gain1 : Gain
  Ground1 : spsGroundLib/Ground  LConnTagsString=a
  Ground2 : spsGroundLib/Ground  LConnTagsString=a
  Ground3 : spsGroundLib/Ground  LConnTagsString=a
  Load Flow Bus1 : spsLoadFlowBusLib/Load Flow Bus  LConnTagsString=a  Phases=single  Connectors=on one side  ID=B5  Vbase=Vhv  Vref=1  Vangle=0  VLF=0.9947  VLFb=1  VLFc=1  angleLF=-30.6  angleLFb=0  angleLFc=0
      settings: SourceProductBaseCode=PS
  Mux : Mux  Inputs=3
  Mux1 : Mux  Inputs=3
  Voltage Measurement1 : spsVoltageMeasurementLib/Voltage Measurement  PhasorSimulation=on  OutputType=Complex  PSBequivalent=0
  Voltage Measurement2 : spsVoltageMeasurementLib/Voltage Measurement  PhasorSimulation=on  OutputType=Complex  PSBequivalent=0
  Voltage Measurement3 : spsVoltageMeasurementLib/Voltage Measurement  PhasorSimulation=on  OutputType=Complex  PSBequivalent=0
  A : PMIOPort  Side=Left
  B : PMIOPort  Port=2  Side=Left
  C : PMIOPort  Port=3  Side=Left
  a : PMIOPort  Port=4  Side=Right
  b : PMIOPort  Port=5  Side=Right
  c : PMIOPort  Port=6  Side=Right
  tag scope: Ig5=global, Vg5=global
  wires:
  Voltage Measurement2/1 -> Mux/3
  Voltage Measurement1/1 -> Mux/2
  Voltage Measurement3/1 -> Mux/1
  Current Measurement3/1 -> Mux1/1
  Current Measurement1/1 -> Mux1/2
  Current Measurement2/1 -> Mux1/3
  Mux/1 -> Gain/1
  Gain/1 -> [Vg5]
  Mux1/1 -> Gain1/1
  Gain1/1 -> [Ig5]
  connections:
  Current Measurement3/RConn1 -- a/RConn1
  Voltage Measurement1/LConn1 -- B/RConn1 -- Current Measurement1/LConn1
  Voltage Measurement2/LConn1 -- C/RConn1 -- Current Measurement2/LConn1
  Voltage Measurement3/LConn1 -- Load Flow Bus1/LConn1 -- A/RConn1 -- Current Measurement3/LConn1
  Current Measurement1/RConn1 -- b/RConn1
  Current Measurement2/RConn1 -- c/RConn1
  Ground3/LConn1 -- Voltage Measurement3/LConn2
  Ground1/LConn1 -- Voltage Measurement1/LConn2
  Ground2/LConn1 -- Voltage Measurement2/LConn2

== system callGAMS/sm_computation/B6 ==
  Current Measurement1 : spsCurrentMeasurementLib/Current Measurement  PhasorSimulation=on  OutputType=Complex  PSBequivalent=0
  Current Measurement2 : spsCurrentMeasurementLib/Current Measurement  PhasorSimulation=on  OutputType=Complex  PSBequivalent=0
  Current Measurement3 : spsCurrentMeasurementLib/Current Measurement  PhasorSimulation=on  OutputType=Complex  PSBequivalent=0
  Gain : Gain
  Gain1 : Gain
  Ground1 : spsGroundLib/Ground  LConnTagsString=a
  Ground2 : spsGroundLib/Ground  LConnTagsString=a
  Ground3 : spsGroundLib/Ground  LConnTagsString=a
  Load Flow Bus1 : spsLoadFlowBusLib/Load Flow Bus  LConnTagsString=a  Phases=single  Connectors=on one side  ID=B6  Vbase=Vhv  Vref=1  Vangle=0  VLF=0.9953  VLFb=1  VLFc=1  angleLF=-30.51  angleLFb=0  angleLFc=0
      settings: SourceProductBaseCode=PS
  Mux : Mux  Inputs=3
  Mux1 : Mux  Inputs=3
  Voltage Measurement1 : spsVoltageMeasurementLib/Voltage Measurement  PhasorSimulation=on  OutputType=Complex  PSBequivalent=0
  Voltage Measurement2 : spsVoltageMeasurementLib/Voltage Measurement  PhasorSimulation=on  OutputType=Complex  PSBequivalent=0
  Voltage Measurement3 : spsVoltageMeasurementLib/Voltage Measurement  PhasorSimulation=on  OutputType=Complex  PSBequivalent=0
  A : PMIOPort  Side=Left
  B : PMIOPort  Port=2  Side=Left
  C : PMIOPort  Port=3  Side=Left
  a : PMIOPort  Port=4  Side=Right
  b : PMIOPort  Port=5  Side=Right
  c : PMIOPort  Port=6  Side=Right
  tag scope: Ig6=global, Vg6=global
  wires:
  Voltage Measurement2/1 -> Mux/3
  Voltage Measurement1/1 -> Mux/2
  Voltage Measurement3/1 -> Mux/1
  Current Measurement3/1 -> Mux1/1
  Current Measurement1/1 -> Mux1/2
  Current Measurement2/1 -> Mux1/3
  Mux/1 -> Gain/1
  Gain/1 -> [Vg6]
  Mux1/1 -> Gain1/1
  Gain1/1 -> [Ig6]
  connections:
  Current Measurement3/RConn1 -- a/RConn1
  Voltage Measurement1/LConn1 -- B/RConn1 -- Current Measurement1/LConn1
  Voltage Measurement2/LConn1 -- C/RConn1 -- Current Measurement2/LConn1
  Voltage Measurement3/LConn1 -- Load Flow Bus1/LConn1 -- A/RConn1 -- Current Measurement3/LConn1
  Current Measurement1/RConn1 -- b/RConn1
  Current Measurement2/RConn1 -- c/RConn1
  Ground3/LConn1 -- Voltage Measurement3/LConn2
  Ground1/LConn1 -- Voltage Measurement1/LConn2
  Ground2/LConn1 -- Voltage Measurement2/LConn2

== system callGAMS/sm_computation/B7 ==
  Current Measurement1 : spsCurrentMeasurementLib/Current Measurement  PhasorSimulation=on  OutputType=Complex  PSBequivalent=0
  Current Measurement2 : spsCurrentMeasurementLib/Current Measurement  PhasorSimulation=on  OutputType=Complex  PSBequivalent=0
  Current Measurement3 : spsCurrentMeasurementLib/Current Measurement  PhasorSimulation=on  OutputType=Complex  PSBequivalent=0
  Gain : Gain
  Gain1 : Gain
  Ground1 : spsGroundLib/Ground  LConnTagsString=a
  Ground2 : spsGroundLib/Ground  LConnTagsString=a
  Ground3 : spsGroundLib/Ground  LConnTagsString=a
  Load Flow Bus1 : spsLoadFlowBusLib/Load Flow Bus  LConnTagsString=a  Phases=single  Connectors=on one side  ID=B7  Vbase=Vhv  Vref=1  Vangle=0  VLF=0.9964  VLFb=1  VLFc=1  angleLF=-29.92  angleLFb=0  angleLFc=0
      settings: SourceProductBaseCode=PS
  Mux : Mux  Inputs=3
  Mux1 : Mux  Inputs=3
  Voltage Measurement1 : spsVoltageMeasurementLib/Voltage Measurement  PhasorSimulation=on  OutputType=Complex  PSBequivalent=0
  Voltage Measurement2 : spsVoltageMeasurementLib/Voltage Measurement  PhasorSimulation=on  OutputType=Complex  PSBequivalent=0
  Voltage Measurement3 : spsVoltageMeasurementLib/Voltage Measurement  PhasorSimulation=on  OutputType=Complex  PSBequivalent=0
  A : PMIOPort  Side=Left
  B : PMIOPort  Port=2  Side=Left
  C : PMIOPort  Port=3  Side=Left
  a : PMIOPort  Port=4  Side=Right
  b : PMIOPort  Port=5  Side=Right
  c : PMIOPort  Port=6  Side=Right
  tag scope: Ig7=global, Vg7=global
  wires:
  Voltage Measurement2/1 -> Mux/3
  Voltage Measurement1/1 -> Mux/2
  Voltage Measurement3/1 -> Mux/1
  Current Measurement3/1 -> Mux1/1
  Current Measurement1/1 -> Mux1/2
  Current Measurement2/1 -> Mux1/3
  Mux/1 -> Gain/1
  Gain/1 -> [Vg7]
  Mux1/1 -> Gain1/1
  Gain1/1 -> [Ig7]
  connections:
  Current Measurement3/RConn1 -- a/RConn1
  Voltage Measurement1/LConn1 -- B/RConn1 -- Current Measurement1/LConn1
  Voltage Measurement2/LConn1 -- C/RConn1 -- Current Measurement2/LConn1
  Voltage Measurement3/LConn1 -- Load Flow Bus1/LConn1 -- A/RConn1 -- Current Measurement3/LConn1
  Current Measurement1/RConn1 -- b/RConn1
  Current Measurement2/RConn1 -- c/RConn1
  Ground3/LConn1 -- Voltage Measurement3/LConn2
  Ground1/LConn1 -- Voltage Measurement1/LConn2
  Ground2/LConn1 -- Voltage Measurement2/LConn2

== system callGAMS/sm_computation/G1 ==
  note: Synchronous Machine Model according to ENTSO-E
  note: Nomenclature (according to IEEE Std 421.1-2007):
      | Efd = Exciter output voltage (generator field voltage)
      | Ifd = Exciter output current (generator field current)
      | Vf = Excitation system stabilizer signal
      | Vfe = Signal proportional to exciter field current
      | Vl = Limiters and protective elements feedback
      | Vr = Regulator output
      | Vs = Power System Stabilizer (PSS) output
      | Vsi = Power System Stabilizer (PSS) inputs (shaft speed, frequency, generator electric power, and others
      | Vt = Generator terminal voltage
      | It = Generator terminal current
      | Vref = Voltage regulator reference signal
      | Vc = terminal voltage transducer output
  Bus Selector : BusSelector  OutputSignals=dw,w,vq,vd,iq,id,Peo,Te
  Exciter System : Subsystem
  Load Flow Bus1 : spsLoadFlowBusLib/Load Flow Bus  LConnTagsString=a  Phases=single  Connectors=on one side  ID=B1_in  Vbase=Vmv  Vref=1  Vangle=0  VLF=1  VLFb=1  VLFc=1  angleLF=0  angleLFb=0  angleLFc=0
      settings: SourceProductBaseCode=PS
  Pm : Constant  Value=0.051106
  Real-Imag to Complex : RealImagToComplex
  Real-Imag to Complex1 : RealImagToComplex
  Ref voltage (p.u) : Constant  Value=1.0
  Scope : Scope
  Snubber : spsThreePhaseParallelRLCLoadLib/Three-Phase Parallel RLC Load  LConnTagsString=A|B|C  Configuration=Y (grounded)  NominalVoltage=Vmv  Vabc=[1e3 1e3 1e3]  Vabcp=[1e3 1e3 1e3]  NominalFrequency=fg  UnbalancedPower=off  ActivePower=S1non*0.05  InductivePower=0  CapacitivePower=0  Pabc=[10e3 9e3 11e3]  QLabc=[100 90 110]  QCabc=[100 90 110]  Pabcp=[10e3 9e3 11e3]  QLabcp=[100 90 110]  QCabcp=[100 90 110]  Measurements=None  LoadType=constant Z
  Speed Governor : Subsystem  mask{R=0.05, T1=0.5, T2=3, T3=10, Dt=0, Vmin=0, Vmax=10, P0=0.051106}
      mask prompts: R "Controller droop (R)"; T1 "Governor time constant (T1)(sec)"; T2 "Turbine derivative time constant (T2)(sec)"; T3 "Turbine delay time constant (T3)(sec)"; Dt "Frictional losses factor (Dt)"; Vmin "Minimum gate limit (Vmin)(p.u)"; Vmax "Maximum gate limit (Vmax)(p.u)"; P0 "Initial power (p.u)"
      mask Display:
      | disp('TGOV')
      | 
      | port_label('input',1,'Pref')
      | port_label('input',2,'dw')
      | 
      | port_label('output',1,'Pm')
  Step : Step  Time=0.2  SampleTime=0
  Switch : Switch  Criteria=u2 > Threshold
  Synchronous Machine pu Standard1 : spsSynchronousMachinepuStandardLib/Synchronous Machine pu Standard  PresetModel=No  MechanicalLoad=Mechanical power Pm  ShowDetailedParameters=on  RotorType=Salient-pole  Units=per unit standard parameters  MeasurementBus=on  NominalParameters=[S1non Vmv fg]  Reactances1=[ 1.81, 0.3, 0.23, 1.76, 0.65, 0.25, 0.15 ]  Reactances2=[1.25 0.333 0.292 1.0 0.292 0.15]  dAxisTimeConstants=Open-circuit  qAxisTimeConstants=Open-circuit  TimeConstants1="[5  0.002  0.002]"  TimeConstants2=[ 8.0, 0.03, 1.0, 0.07 ]  TimeConstants3="[  4.49  0.0681  0.0513  ]"  TimeConstants4=[ 8.0, 0.03, 0.3371, 0.0295 ]  TimeConstants5=[ 1.01, 0.053, 0.1 ]  TimeConstants6=[ 1.3201, 0.023, 1.0, 0.07 ]  TimeConstants7=[0.012 0.003 0.003]  TimeConstants8=[ 1.3201, 0.0231, 0.3371, 0.0295 ]  StatorResistance=0.01  Mechanical=[5 0 2]  PolePairs=20  InitialConditions=[0 -87.0786 0.0510815 0.0510815 0.0510815 -0.412798 -120.413 119.587 1.00292]  SetSaturation=off  Saturation=[0.6404,0.7127,0.8441,0.9214,0.9956,1.082,1.19,1.316,1.457;0.7,0.7698,0.8872,0.9466,0.9969,1.046,1.1,1.151,1.201]  LoadFlowParameters=[1,0,0,0,0]  TsPowergui=0  TsBlock=-1  IterativeModel=Trapezoidal non iterative  IterativeDiscreteModel=Trapezoidal non iterative  BusType=swing  Pref=0  Qref=0  Qmin=-inf  Qmax=inf  PLF=0  QLF=0
      settings: SourceProductBaseCode=PS
  Three-Phase Transformer (Two Windings)1 : spsThreePhaseTransformerTwoWindingsLib/Three-Phase Transformer (Two Windings)  Winding1Connection=Delta (D11)  Winding2Connection=Yg  CoreType=Three single-phase transformers  SetSaturation=off  Hysteresis=off  DataFile='hysteresis'  SetInitialFlux=off  Measurements=None  UNITS=pu  NominalPower=[S1non , fg]  Winding1=[Vmv 0.00125 0.05]  Winding2=[Vhv 0.00125 0.05]  Rm=5000  Lm=5000  L0=0.5  Saturation=[ 0,0 ; 0.0024,1.2 ; 1.0,1.52 ]  InitialFluxes=[ 0.8 , -0.8 , 0.7 ]  BreakLoop=off  DiscreteSolver=Trapezoidal iterative  DataType=off  TransfoNumber=1
  A : PMIOPort  Side=Right
  B : PMIOPort  Port=2  Side=Right
  C : PMIOPort  Port=3  Side=Right
  tag scope: Pe1=global, Te1=global, wm1=global
  wires:
  Bus Selector/1 -> Speed Governor/2(dw), Exciter System/1(<dw>)  "<dw>"
  Bus Selector/4 -> Real-Imag to Complex/2  "<vd>"
  Bus Selector/3 -> Real-Imag to Complex/1  "<vq>"
  Bus Selector/5 -> Real-Imag to Complex1/1  "<iq>"
  Bus Selector/6 -> Real-Imag to Complex1/2  "<id>"
  Real-Imag to Complex/1 -> Exciter System/3(Vt)
  Real-Imag to Complex1/1 -> Exciter System/4(It)
  Bus Selector/8 -> [Te1]  "<Te>"
  Exciter System/1(Efd) -> Synchronous Machine pu Standard1/2
  Synchronous Machine pu Standard1/1 -> Bus Selector/1
  Pm/1 -> Speed Governor/1(RefL)
  Bus Selector/2 -> [wm1]  "<w>"
  Bus Selector/7 -> [Pe1], Scope/1, Exciter System/5(<Peo>)  "<Peo>"
  Ref voltage (p.u)/1 -> Exciter System/2(Vref)
  Speed Governor/1(Pm) -> Switch/1
  Step/1 -> Switch/2
  [Pe1] -> Switch/3
  Switch/1 -> Synchronous Machine pu Standard1/1
  connections:
  Synchronous Machine pu Standard1/RConn1 -- Load Flow Bus1/LConn1 -- Three-Phase Transformer (Two Windings)1/LConn1 -- Snubber/LConn1
  Synchronous Machine pu Standard1/RConn3 -- Three-Phase Transformer (Two Windings)1/LConn3 -- Snubber/LConn3
  Synchronous Machine pu Standard1/RConn2 -- Three-Phase Transformer (Two Windings)1/LConn2 -- Snubber/LConn2
  Three-Phase Transformer (Two Windings)1/RConn1 -- A/RConn1
  Three-Phase Transformer (Two Windings)1/RConn2 -- B/RConn1
  Three-Phase Transformer (Two Windings)1/RConn3 -- C/RConn1
